simulink model "CaseStudyII_9_Bus"  (R2020a)
settings: Solver=FixedStepAuto  StartTime=0.0  StopTime=Tend  FixedStep=T_s_power  MaxStep=5.0E-5  RelTol=1e-3
values from neighbouring files (symbols this model uses):
  B_s46 = b_s46*Cb    (= 9.5071761847e-07)    [Data_CaseStudyI.m]    (also in Data_CaseStudyII.m; Data_InitialSystem.m)
  B_s54 = b_s54*Cb    (= 1.05902722057e-06)    [Data_CaseStudyI.m]    (also in Data_CaseStudyII.m; Data_InitialSystem.m)
  B_s69 = b_s69*Cb    (= 2.15415764185e-06)    [Data_CaseStudyI.m]    (also in Data_CaseStudyII.m; Data_InitialSystem.m)
  B_s75 = b_s75*Cb    (= 1.84126323577e-06)    [Data_CaseStudyI.m]    (also in Data_CaseStudyII.m; Data_InitialSystem.m)
  B_s87 = b_s87*Cb    (= 8.96562817417e-07)    [Data_CaseStudyI.m]    (also in Data_CaseStudyII.m; Data_InitialSystem.m)
  B_s98 = b_s98*Cb    (= 1.25759482443e-06)    [Data_CaseStudyI.m]    (also in Data_CaseStudyII.m; Data_InitialSystem.m)
  C_dc_DVPP_1_2 = 0.008*(n_DVPP_1_2)    (= 0.8)    [Data_CaseStudyI.m]    (also in Data_CaseStudyII.m)
  C_dc_DVPP_1_3 = 0.008*(n_DVPP_1_3)    (= 0.4)    [Data_CaseStudyI.m]    (also in Data_CaseStudyII.m)
  C_dc_DVPP_3_1 = 0.008*(n_DVPP_3_1)    (= 1.128)    [Data_CaseStudyII.m]
  C_dc_DVPP_3_2 = 0.008*(n_DVPP_3_2)    (= 0.848)    [Data_CaseStudyII.m]
  C_dc_DVPP_3_3 = 0.008*(n_DVPP_3_3)    (= 1.28)    [Data_CaseStudyII.m]
  Dp_DVPP_3_pu = 1/dp_DVPP_3    (= 33.3333333333)    [Data_CaseStudyII.m]
  Dq1_DVPP_3_pu = 100    [Data_CaseStudyII.m]
  fb = 50    [Data_CaseStudyI.m]    (also in Data_CaseStudyII.m; Data_InitialSystem.m)
  HGov_dyn = HGov_delay*H_tr_droop    [Data_CaseStudyI.m]    (also in Data_CaseStudyII.m; Data_InitialSystem.m)
  HTurb_tot = H_water_way    [Data_CaseStudyI.m]    (also in Data_CaseStudyII.m; Data_InitialSystem.m)
  I_m_DVPP_1_2 = 2/3*Sb_DVPP_1_2/V_m_DVPP_1_2    [Data_CaseStudyI.m]    (also in Data_CaseStudyII.m)
  I_m_DVPP_1_3 = 2/3*Sb_DVPP_1_3/V_m_DVPP_1_3    [Data_CaseStudyI.m]    (also in Data_CaseStudyII.m)
  I_m_DVPP_3_1 = 2/3*Sb_DVPP_3_1/V_m_DVPP_3_1    [Data_CaseStudyII.m]
  I_m_DVPP_3_2 = 2/3*Sb_DVPP_3_2/V_m_DVPP_3_2    [Data_CaseStudyII.m]
  I_m_DVPP_3_3 = 2/3*Sb_DVPP_3_3/V_m_DVPP_3_3    [Data_CaseStudyII.m]
  i_star_max = 1.3    [Data_CaseStudyI.m]    (also in Data_CaseStudyII.m)
  iabc_DVPP_1_2_0 = T0*idq0_DVPP_1_2    [Data_CaseStudyI.m]    (also in Data_CaseStudyII.m)
  iabc_DVPP_1_3_0 = T0*idq0_DVPP_1_3    [Data_CaseStudyI.m]    (also in Data_CaseStudyII.m)
  iabc_DVPP_3_1_0 = T0*idq0_DVPP_3_1    [Data_CaseStudyII.m]
  iabc_DVPP_3_2_0 = T0*idq0_DVPP_3_2    [Data_CaseStudyII.m]
  iabc_DVPP_3_3_0 = T0*idq0_DVPP_3_3    [Data_CaseStudyII.m]
  K2_DVPP_1 = [-0.0221795494247 -1.60799665656 0.160449825826 -2.94803557381 -11.8081988371 -9.75170960256 0.00463021906909 -49.1667298155]    [ControlGains_DVPP1.mat]
  K3_DVPP_1 = [-0.0591512752956 -1.61493903379 -27.2946107927 -16.2119211358 -14.3657419818 2.05688388773 -2.27328406162 0.146700393037 -150.920793597]    [ControlGains_DVPP1.mat]
  k_dc_DVPP_1_2 = eta_DVPP_1_2/(Vdc_n_DVPP_1_2*m_p_DVPP_1_2)    [Data_CaseStudyI.m]    (also in Data_CaseStudyII.m)
  k_dc_DVPP_1_3 = eta_DVPP_1_3/(Vdc_n_DVPP_1_3*m_p_DVPP_1_3)    [Data_CaseStudyI.m]    (also in Data_CaseStudyII.m)
  k_dc_DVPP_3_1 = eta_DVPP_3_1/(Vdc_n_DVPP_3_1*m_p_DVPP_3_1)    [Data_CaseStudyII.m]
  k_dc_DVPP_3_2 = eta_DVPP_3_2/(Vdc_n_DVPP_3_2*m_p_DVPP_3_2)    [Data_CaseStudyII.m]
  k_dc_DVPP_3_3 = eta_DVPP_3_3/(Vdc_n_DVPP_3_3*m_p_DVPP_3_3)    [Data_CaseStudyII.m]
  ki_i_pu = 1.19    [Data_CaseStudyI.m]    (also in Data_CaseStudyII.m)
  ki_pll = 1700    [Data_CaseStudyI.m]    (also in Data_CaseStudyII.m)
  ki_q_pu = 0.005    [Data_CaseStudyI.m]    (also in Data_CaseStudyII.m)
  kp_i_pu = 0.73    [Data_CaseStudyI.m]    (also in Data_CaseStudyII.m)
  kp_pll = 150    [Data_CaseStudyI.m]    (also in Data_CaseStudyII.m)
  kp_q_pu = 0.05    [Data_CaseStudyI.m]    (also in Data_CaseStudyII.m)
  L1_DVPP_1_2_pu = 0.0186/m_DVPP_1_2    (= 0.000372)    [Data_CaseStudyI.m]    (also in Data_CaseStudyII.m)
  L1_DVPP_1_3_pu = 0.0186/m_DVPP_1_3    (= 0.000744)    [Data_CaseStudyI.m]    (also in Data_CaseStudyII.m)
  L1_DVPP_3_1_pu = 0.0186/m_DVPP_3_1    (= 0.000263829787234)    [Data_CaseStudyII.m]
  L1_DVPP_3_2_pu = 0.0186/m_DVPP_3_2    (= 0.000350943396226)    [Data_CaseStudyII.m]
  L1_DVPP_3_3_pu = 0.0186/m_DVPP_3_3    (= 0.0002325)    [Data_CaseStudyII.m]
  l1_MVHV1 = 0    [Data_CaseStudyI.m]    (also in Data_CaseStudyII.m; Data_InitialSystem.m)
  l1_MVHV2 = 0    [Data_CaseStudyI.m]    (also in Data_CaseStudyII.m; Data_InitialSystem.m)
  l1_MVHV3 = 0    [Data_CaseStudyI.m]    (also in Data_CaseStudyII.m; Data_InitialSystem.m)
  L2_DVPP_1_2_pu = L1_DVPP_1_2_pu    (= 0.000372)    [Data_CaseStudyI.m]    (also in Data_CaseStudyII.m)
  L2_DVPP_1_3_pu = L1_DVPP_1_3_pu    (= 0.000744)    [Data_CaseStudyI.m]    (also in Data_CaseStudyII.m)
  L2_DVPP_3_1_pu = L1_DVPP_3_1_pu    (= 0.000263829787234)    [Data_CaseStudyII.m]
  L2_DVPP_3_2_pu = L1_DVPP_3_2_pu    (= 0.000350943396226)    [Data_CaseStudyII.m]
  L2_DVPP_3_3_pu = L1_DVPP_3_3_pu    (= 0.0002325)    [Data_CaseStudyII.m]
  l2_MVHV1 = l_s14    (= 0.0576)    [Data_CaseStudyI.m]    (also in Data_CaseStudyII.m; Data_InitialSystem.m)
  l2_MVHV2 = l_s72    (= 0.0625)    [Data_CaseStudyI.m]    (also in Data_CaseStudyII.m; Data_InitialSystem.m)
  l2_MVHV3 = l_s39    (= 0.0586)    [Data_CaseStudyI.m]    (also in Data_CaseStudyII.m; Data_InitialSystem.m)
  l_f_DVPP_1_2 = L_f_DVPP_1_2*w_b/Zb_DVPP_1_2    [Data_CaseStudyI.m]    (also in Data_CaseStudyII.m)
  L_f_DVPP_1_2 = (1/(n_DVPP_1_2))*600*10^-6    (= 6e-06)    [Data_CaseStudyI.m]    (also in Data_CaseStudyII.m)
  l_f_DVPP_1_3 = L_f_DVPP_1_3*w_b/Zb_DVPP_1_3    [Data_CaseStudyI.m]    (also in Data_CaseStudyII.m)
  L_f_DVPP_1_3 = (1/(n_DVPP_1_3))*600*10^-6    (= 1.2e-05)    [Data_CaseStudyI.m]    (also in Data_CaseStudyII.m)
  l_f_DVPP_3_1 = L_f_DVPP_3_1*w_b/Zb_DVPP_3_1    [Data_CaseStudyII.m]
  L_f_DVPP_3_1 = (1/(n_DVPP_3_1))*600*10^-6    (= 4.25531914894e-06)    [Data_CaseStudyII.m]
  l_f_DVPP_3_2 = L_f_DVPP_3_2*w_b/Zb_DVPP_3_2    [Data_CaseStudyII.m]
  L_f_DVPP_3_2 = (1/(n_DVPP_3_2))*600*10^-6    (= 5.66037735849e-06)    [Data_CaseStudyII.m]
  l_f_DVPP_3_3 = L_f_DVPP_3_3*w_b/Zb_DVPP_3_3    [Data_CaseStudyII.m]
  L_f_DVPP_3_3 = (1/(n_DVPP_3_3))*600*10^-6    (= 3.75e-06)    [Data_CaseStudyII.m]
  L_s46 = l_s46*Lb    (= 0.154915055408)    [Data_CaseStudyI.m]    (also in Data_CaseStudyII.m; Data_InitialSystem.m)
  L_s54 = l_s54*Lb    (= 0.143128040323)    [Data_CaseStudyI.m]    (also in Data_CaseStudyII.m; Data_InitialSystem.m)
  L_s69 = l_s69*Lb    (= 0.286256080645)    [Data_CaseStudyI.m]    (also in Data_CaseStudyII.m; Data_InitialSystem.m)
  L_s75 = l_s75*Lb    (= 0.271101346964)    [Data_CaseStudyI.m]    (also in Data_CaseStudyII.m; Data_InitialSystem.m)
  L_s87 = l_s87*Lb    (= 0.12123786945)    [Data_CaseStudyI.m]    (also in Data_CaseStudyII.m; Data_InitialSystem.m)
  L_s98 = l_s98*Lb    (= 0.16973301723)    [Data_CaseStudyI.m]    (also in Data_CaseStudyII.m; Data_InitialSystem.m)
  LPV_K1_DVPP_3 = [0.014519129833 -1.24253756746e-17 -0.00331576987938 -1.41950397655e-17 -0.00331577010739 -1.6423216922e-19 0.0145191298795 1.47256053017e-18 1.92456501739e-17 0.00968260817745 7.5102914291e-19 0.0096826081765 ... (80 elements, 8x10)]    [ControlGains_DVPP3_LPV.mat]
  LPV_K2_DVPP_3 = [0.0299413265511 -2.72480441208e-16 -0.00563144274341 -6.63344905835e-17 -0.00563144273182 -1.08918556426e-16 0.0299413268326 -1.32404731664e-16 -4.78559537004e-17 -0.00914230292149 -8.50409089014e-21 -0.00914230292147 ... (80 elements, 8x10)]    [ControlGains_DVPP3_LPV.mat]
  LPV_K3_DVPP_3 = [-0.0173301370849 5.00398589077e-17 -0.0636125194304 3.31757376688e-17 -0.0636125164794 5.41726806116e-17 -0.017330137145 2.43427565927e-17 -0.0400570975704 -5.68753124238e-17 -0.0574012283733 2.45717741258e-17 ... (192 elements, 16x12)]    [ControlGains_DVPP3_LPV.mat]
  Mp_DVPP_3_pu = 13    [Data_CaseStudyII.m]
  P_L = pL*Sb    (= 300000000)    [Data_CaseStudyI.m]    (also in Data_CaseStudyII.m; Data_InitialSystem.m)
  p_set_bus1 = P_set_bus1/SbSG1    (= 0.731707317073)    [Data_CaseStudyI.m]    (also in Data_CaseStudyII.m; Data_InitialSystem.m)
  p_set_bus2 = P_set_bus2/SbSG2    (= 0.756707317073)    [Data_CaseStudyI.m]    (also in Data_CaseStudyII.m; Data_InitialSystem.m)
  Pb_DVPP_3_1 = 37e6    (= 37000000)    [Data_CaseStudyII.m]
  Pb_DVPP_3_2 = 28e6    (= 28000000)    [Data_CaseStudyII.m]
  Pb_DVPP_3_3 = 0e6    (= 0)    [Data_CaseStudyII.m]
  pset_DVPP_1_1 = P_set_bus1/SbSG1    (= 0.731707317073)    [Data_CaseStudyI.m]    (also in Data_CaseStudyII.m)
  pset_DVPP_1_2 = 0    [Data_CaseStudyI.m]    (also in Data_CaseStudyII.m)
  pset_DVPP_1_3 = 0    [Data_CaseStudyI.m]    (also in Data_CaseStudyII.m)
  pset_DVPP_3_1 = (0.6*P_set_bus3)/Sb_DVPP_3_1    (= 0.398546964193)    [Data_CaseStudyII.m]
  pset_DVPP_3_2 = (0.4*P_set_bus3)/Sb_DVPP_3_2    (= 0.353428439945)    [Data_CaseStudyII.m]
  pset_DVPP_3_3 = 0    [Data_CaseStudyII.m]
  Q_L = qL*Sb    (= 82500000)    [Data_CaseStudyI.m]    (also in Data_CaseStudyII.m; Data_InitialSystem.m)
  qset_DVPP_1_2 = 0    [Data_CaseStudyI.m]    (also in Data_CaseStudyII.m)
  qset_DVPP_1_3 = 0    [Data_CaseStudyI.m]    (also in Data_CaseStudyII.m)
  qset_DVPP_3_1 = 0    [Data_CaseStudyII.m]
  qset_DVPP_3_2 = 0    [Data_CaseStudyII.m]
  qset_DVPP_3_3 = 0    [Data_CaseStudyII.m]
  R1_DVPP_1_2_pu = 0.00734/m_DVPP_1_2    (= 0.0001468)    [Data_CaseStudyI.m]    (also in Data_CaseStudyII.m)
  R1_DVPP_1_3_pu = 0.00734/m_DVPP_1_3    (= 0.0002936)    [Data_CaseStudyI.m]    (also in Data_CaseStudyII.m)
  R1_DVPP_3_1_pu = 0.00734/m_DVPP_3_1    (= 0.000104113475177)    [Data_CaseStudyII.m]
  R1_DVPP_3_2_pu = 0.00734/m_DVPP_3_2    (= 0.000138490566038)    [Data_CaseStudyII.m]
  R1_DVPP_3_3_pu = 0.00734/m_DVPP_3_3    (= 9.175e-05)    [Data_CaseStudyII.m]
  r1_MVHV1 = 1e-6    (= 1e-06)    [Data_CaseStudyI.m]    (also in Data_CaseStudyII.m; Data_InitialSystem.m)
  r1_MVHV2 = 1e-6    (= 1e-06)    [Data_CaseStudyI.m]    (also in Data_CaseStudyII.m; Data_InitialSystem.m)
  r1_MVHV3 = 1e-6    (= 1e-06)    [Data_CaseStudyI.m]    (also in Data_CaseStudyII.m; Data_InitialSystem.m)
  R2_DVPP_1_2_pu = R1_DVPP_1_2_pu    (= 0.0001468)    [Data_CaseStudyI.m]    (also in Data_CaseStudyII.m)
  R2_DVPP_1_3_pu = R1_DVPP_1_3_pu    (= 0.0002936)    [Data_CaseStudyI.m]    (also in Data_CaseStudyII.m)
  R2_DVPP_3_1_pu = R1_DVPP_3_1_pu    (= 0.000104113475177)    [Data_CaseStudyII.m]
  R2_DVPP_3_2_pu = R1_DVPP_3_2_pu    (= 0.000138490566038)    [Data_CaseStudyII.m]
  R2_DVPP_3_3_pu = R1_DVPP_3_3_pu    (= 9.175e-05)    [Data_CaseStudyII.m]
  r2_MVHV1 = 1e-6    (= 1e-06)    [Data_CaseStudyI.m]    (also in Data_CaseStudyII.m; Data_InitialSystem.m)
  r2_MVHV2 = 1e-6    (= 1e-06)    [Data_CaseStudyI.m]    (also in Data_CaseStudyII.m; Data_InitialSystem.m)
  r2_MVHV3 = 1e-6    (= 1e-06)    [Data_CaseStudyI.m]    (also in Data_CaseStudyII.m; Data_InitialSystem.m)
  R_dc_DVPP_1_2 = (Vdc_n_DVPP_1_2/(0.05*(Sb_DVPP_1_2)/Vdc_n_DVPP_1_2))    [Data_CaseStudyI.m]    (also in Data_CaseStudyII.m)
  R_dc_DVPP_1_3 = (Vdc_n_DVPP_1_3/(0.05*(Sb_DVPP_1_3)/Vdc_n_DVPP_1_3))    [Data_CaseStudyI.m]    (also in Data_CaseStudyII.m)
  R_dc_DVPP_3_1 = (Vdc_n_DVPP_3_1/(0.05*(Sb_DVPP_3_1)/Vdc_n_DVPP_3_1))    [Data_CaseStudyII.m]
  R_dc_DVPP_3_2 = (Vdc_n_DVPP_3_2/(0.05*(Sb_DVPP_3_2)/Vdc_n_DVPP_3_2))    [Data_CaseStudyII.m]
  R_dc_DVPP_3_3 = (Vdc_n_DVPP_3_3/(0.05*(Sb_DVPP_3_3)/Vdc_n_DVPP_3_3))    [Data_CaseStudyII.m]
  r_f_DVPP_1_2 = R_f_DVPP_1_2/Zb_DVPP_1_2    [Data_CaseStudyI.m]    (also in Data_CaseStudyII.m)
  R_f_DVPP_1_2 = 0.02/n_DVPP_1_2    (= 0.0002)    [Data_CaseStudyI.m]    (also in Data_CaseStudyII.m)
  r_f_DVPP_1_3 = R_f_DVPP_1_3/Zb_DVPP_1_3    [Data_CaseStudyI.m]    (also in Data_CaseStudyII.m)
  R_f_DVPP_1_3 = 0.02/n_DVPP_1_3    (= 0.0004)    [Data_CaseStudyI.m]    (also in Data_CaseStudyII.m)
  r_f_DVPP_3_1 = R_f_DVPP_3_1/Zb_DVPP_3_1    [Data_CaseStudyII.m]
  ... (+104 more)
undefined symbols (not defined in the file or in its folder): A, B, C, Continuous, Dd, Efd0, gcbh, i_dc, Ka, Kf, p2set, SbSM2, sps_rtmsupport, spsST1AModel, Ta, Tb, Tb1, Tc, Tc1, Tf, VA0, VAmax, VAmin, VImax, VImin, VRmax, VRmin
libraries: powerlib x95, powerlib_meascontrol x41, cstblocks x15, sps_avr x1, simulink_extras x1, simulink x1
(part 5 of 5)

== system CaseStudyII_9_Bus/Supercapacitor/Power Controllers/Reactive Power Controller PI-droop control ==
  Q_abc : Inport
  Qset : Inport  Port=2
  Gain : Gain  Gain=kp_q_pu
  Gain1 : Gain  Gain=ki_q_pu
  Integrator1 : Integrator  InitialCondition=xq0_DVPP_1_3_pu
  Sum : Sum  Inputs=-+
  Sum1 : Sum
  i_star_q : Outport
  wires:
  Q_abc/1 -> Sum/2
  Qset/1 -> Sum/1
  Sum/1 -> Integrator1/1, Gain/1
  Gain/1 -> Sum1/1
  Gain1/1 -> Sum1/2
  Integrator1/1 -> Gain1/1
  Sum1/1 -> i_star_q/1

== system CaseStudyII_9_Bus/Synchronous Machine 2 reheat steam turbine/ST1A Excitation System/Model ==
  note: Efd0
  note: Efd0
  note: VA0/Ka
  note: VA0/Ka
  note: Vt.VRmin
  note: VA0/Ka
  note: Efd0
  note: 0
  note: Vt0
  note: Vt.VRmax-Kc.Ifd
  note: Main Regulator
      | Ka/(Ta.s+1)
  note: VImax
  note: Initial values are shown in blue
  note: Vt0
  note: __
      |              /
      |           /
      |         /
      |       /
      | __/
  note: Limits VImin, VImax
  note: VAmax
  note: VAmin
  note: VA0/Ka
  note: KLR*(Ifd-ILR)
  note: VA0=Efd0+KLR*(Ifd-ILR)
  note: VA0
  note: Vt0
  Vref : Inport
  Vt : Inport  Port=2
  Ifd : Inport  Port=3
  Vstab : Inport  Port=4
  Damping Filter Kf.s/(Tf.s+1) : Subsystem  mask(Transfer Function with Initial Outputs){N=[Kf 0], D=[Tf 1], Y0=0, U0=Efd0}
      mask prompts: N "Numerator:"; D "Denominator:"; Y0 "Initial output:"; U0 "Initial input:"
      mask help: Vector expressions for numerator, and denominator. Coefficients are in descending powers of s.
      mask init:
      | [A,B,C,Dd]=tf2ss(N,D);
      | if (isempty(Y0));
      |     [m,n]=size(C);
      |     Y0=zeros(1,m); 
      | end; 
      | if (isempty(U0));
      |     [m,p]=size(B);
      |     U0=zeros(1,p);
      | end;
      | X0=getxo(A,B,C,Dd,U0,Y0,0);
      mask Help: Specify the initial output for the transfer function.  An optimization routine attempts to determine the appropriate initial states so that the specified initial output is achieved.  For more details, see the m-file getxo.m
      mask Display: dpoly(N,D,'s')
  ILR : Constant  Value=ILR
  KLR : Gain  Gain=KLR  SaturateOnIntegerOverflow=on  OutDataTypeStr=Inherit: Same as input  ParamDataTypeStr=Inherit: Same as input
  Low Pass Filter 1/(Tr.s+1) : simulink_extras/Additional Linear/Transfer Fcn (with initial outputs)  N=1  D=[Tr 1]  Y0=Vt0  U0=Vt0
  Subsystem : Subsystem
      mask Display: plot([0.15 0.85],[.5 .5],[.5 .5],[0.05 0.95],0.15+0.7*[0 .25 .75 1],0.05+0.9*[.25 .25 .75 .75]);
  Subtract : Sum  Inputs=+-
  Sum : Sum  Inputs=++-+-  InputSameDT=on  SaturateOnIntegerOverflow=on  OutDataTypeStr=Inherit: Same as first input
  Sum1 : Sum  Inputs=|+-  InputSameDT=on  SaturateOnIntegerOverflow=on  OutDataTypeStr=Inherit: Same as first input
  Sum2 : Sum  Inputs=|+-  InputSameDT=on  SaturateOnIntegerOverflow=on  OutDataTypeStr=Inherit: Same as first input
  Transient Gain Reduction (Tc.s+1).(Tc1.s+1) ----------------------- (Tb.s+1).(Tb1.s+1) : Subsystem  mask(Transfer Function with Initial Outputs){N=[Tc*Tc1 Tc+Tc1 1], D=[Tb*Tb1 Tb+Tb1 1], Y0=VA0/Ka, U0=VA0/Ka}
      mask prompts: N "Numerator:"; D "Denominator:"; Y0 "Initial output:"; U0 "Initial input:"
      mask help: Vector expressions for numerator, and denominator. Coefficients are in descending powers of s.
      mask init:
      | [A,B,C,Dd]=tf2ss(N,D);if (isempty(Y0));[m,n]=size(A);X0=zeros(1,m); end; if (isempty(U0));[m,p]=size(B);U0=zeros(1,p);end;
      |  if isempty(A),  X0=[]; else ,X0=getxo(A,B,C,Dd,U0,Y0,0); end
      mask Help: Specify the initial output for the transfer function.  An optimization routine attempts to determine the appropriate initial states so that the specified initial output is achieved.  For more details, see the m-file getxo.m
      mask Display: dpoly(N,D,'s')
  VA0/Ka : Constant  Value=VA0/Ka
  VImin : Saturate  UpperLimit=VImax  LowerLimit=VImin
  VImin2 : Saturate  UpperLimit=inf  LowerLimit=0
  Vaminmax : Subsystem  mask{Ka=Ka, Ta=Ta, VAminmax=[VAmin VAmax], X0=VA0}
      mask prompts: Ka "Voltage regulator gain Ka:"; Ta "Voltage regulator time constant Ta(s):"; VAminmax "Voltage regulator internal limits [VAmin(pu) VAmax(pu)]:"; X0 "Initial conditions:"
      mask init:
      | VAmin=VAminmax(1);VAmax=VAminmax(2);
      mask Display: dpoly([Ka],[Ta 1],'s')
  Efd : Outport
  wires:
  Ifd/1 -> Sum1/1, Subsystem/3(Ifd)
  Subsystem/1(Efd1) -> Efd/1  "Efd"
  Vt/1 -> Low Pass Filter 1/(Tr.s+1)/1  "Vt"
  Vaminmax/1(y) -> Sum2/1  "VA"
  Sum/1 -> VImin/1
  Sum1/1 -> KLR/1
  ILR/1 -> Sum1/2
  Sum2/1 -> Damping Filter Kf.s/(Tf.s+1)/1(In1), Subsystem/1(Efd)  "Efd"
  Transient Gain Reduction (Tc.s+1).(Tc1.s+1) ----------------------- (Tb.s+1).(Tb1.s+1)/1(Out1) -> Vaminmax/1(u)
  KLR/1 -> VImin2/1
  VA0/Ka/1 -> Sum/2
  Low Pass Filter 1/(Tr.s+1)/1 -> Subtract/2, Subsystem/2(Vt)  "Vt"
  VImin2/1 -> Sum2/2
  Damping Filter Kf.s/(Tf.s+1)/1(Out1) -> Sum/5  "Vf"
  VImin/1 -> Transient Gain Reduction (Tc.s+1).(Tc1.s+1) ----------------------- (Tb.s+1).(Tb1.s+1)/1(In1)  "VI"
  Vstab/1 -> Sum/4
  Vref/1 -> Subtract/1
  Subtract/1 -> Sum/1

== system CaseStudyII_9_Bus/Wind /PLL/Subsystem ==
  Vabc : Inport  PortDimensions=3
  Constant : Constant  Value=2*pi*50
  Demux2 : Demux  Outputs=3
  Divide : Product  Inputs=/*
  First-Order Filter : powerlib_meascontrol/Filters/First-Order Filter  FilterType=Lowpass  Tc=0.081  Ts=0  Initialize=on  Vac_Init=[0, 0, fb]  Vdc_Init=0  PlotResponse=off  FreqRange="[0,  200,  1]"
  Gain : Gain  Gain=kp_pll
  Gain1 : Gain  Gain=ki_pll
  Gain10 : Gain  Gain=1/2/pi  SaturateOnIntegerOverflow=on  OutDataTypeStr=Inherit: Same as input  ParamDataTypeStr=Inherit: Same as input
  Integrator : Integrator
  Integrator1 : Integrator  InitialCondition=xpll0_pu
  Memory : Memory  InitialCondition=fb
  Selector : Selector  InputPortWidth=3  IndexOptions=Index vector (dialog)  Indices=2  OutputSizes=1
  Sqrt2 : Sqrt  SaturateOnIntegerOverflow=on
  Sum : Sum
  Sum1 : Sum  Inputs=++|
  Sum2 : Sum  Inputs=+++  InputSameDT=on  SaturateOnIntegerOverflow=on  OutDataTypeStr=Inherit: Same as first input
  abc to dq0 : powerlib_meascontrol/Transformations/abc to dq0  Alignment=90 degrees behind phase A axis
      settings: SourceProductBaseCode=MT,PS
  d²2 : Product  InputSameDT=on  RndMeth=Zero  SaturateOnIntegerOverflow=on  OutDataTypeStr=Inherit: Same as first input
  q²4 : Product  InputSameDT=on  RndMeth=Zero  SaturateOnIntegerOverflow=on  OutDataTypeStr=Inherit: Same as first input
  q²5 : Product  InputSameDT=on  RndMeth=Zero  SaturateOnIntegerOverflow=on  OutDataTypeStr=Inherit: Same as first input
  Freq : Outport  VectorParamsAs1DForOutWhenUnconnected=off
  wt : Outport  Port=2  VectorParamsAs1DForOutWhenUnconnected=off
  wires:
  Vabc/1 -> abc to dq0/1
  Integrator/1 -> wt/1, abc to dq0/2
  Memory/1 -> Freq/1
  Gain/1 -> Sum/1
  Gain1/1 -> Sum/2
  Integrator1/1 -> Gain1/1
  Demux2/1 -> d²2/1, d²2/2  "d"
  d²2/1 -> Sum2/1
  Demux2/3 -> q²5/1, q²5/2  "0"
  Demux2/2 -> q²4/1, q²4/2  "q"
  Sqrt2/1 -> Divide/1
  Sum2/1 -> Sqrt2/1
  q²5/1 -> Sum2/3
  abc to dq0/1 -> Demux2/1, Selector/1
  q²4/1 -> Sum2/2
  Selector/1 -> Divide/2  "Vq"
  Divide/1 -> Integrator1/1, Gain/1
  Gain10/1 -> First-Order Filter/1
  First-Order Filter/1 -> Memory/1
  Constant/1 -> Sum1/1
  Sum/1 -> Sum1/2  "W"
  Sum1/1 -> Integrator/1, Gain10/1  "W"

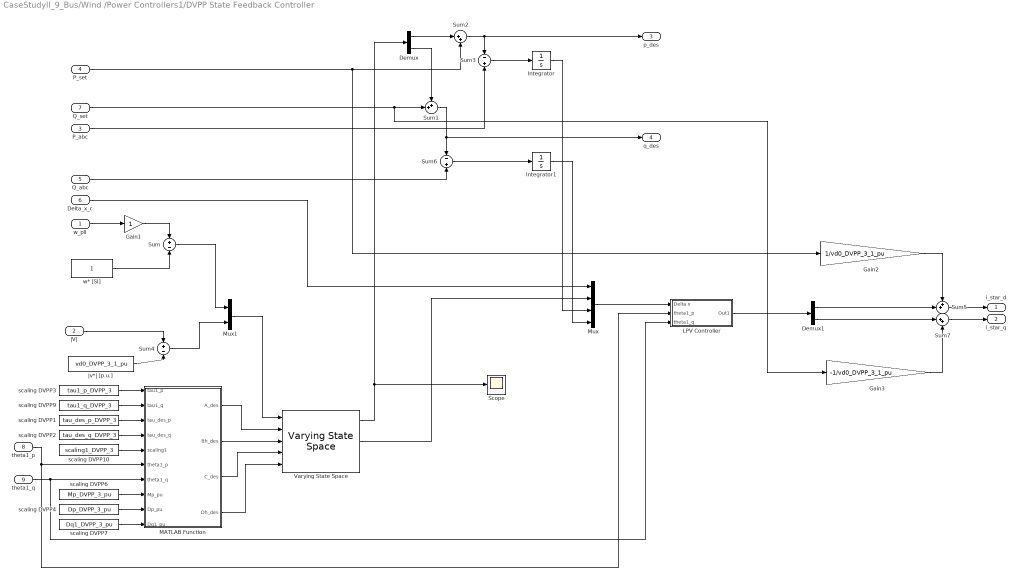
== system CaseStudyII_9_Bus/Wind /Power Controllers1/DVPP State Feedback Controller ==
  w_pll : Inport
  "|V| " : Inport  Port=2
  P_abc : Inport  Port=3
  P_set : Inport  Port=4
  Q_abc : Inport  Port=5
  Delta_x_c : Inport  Port=6
  Q_set : Inport  Port=7
  theta1_p : Inport  Port=8
  theta1_q : Inport  Port=9
  Demux : Demux  Outputs=2
  Demux1 : Demux  Outputs=2
  Gain1 : Gain
  Gain2 : Gain  Gain=1/vd0_DVPP_3_1_pu
  Gain3 : Gain  Gain=-1/vd0_DVPP_3_1_pu
  Integrator : Integrator
  Integrator1 : Integrator
  LPV Controller : Subsystem
  MATLAB Function : MATLAB Function  TreatAsAtomicUnit=on
  Mux : Mux
  Mux1 : Mux  Inputs=2
  Scope : Scope
  Sum : Sum  Inputs=+-
  Sum1 : Sum  Inputs=++|
  Sum2 : Sum  Inputs=|++
  Sum3 : Sum  Inputs=-+
  Sum4 : Sum  Inputs=+-
  Sum5 : Sum  Inputs=++|
  Sum6 : Sum  Inputs=-+
  Sum7 : Sum  Inputs=|++
  Varying State Space : cstblocks/Linear Parameter Varying/Varying State Space  x0=0  xNames=''  OutputX=on  OutputDX=on
  scaling DVPP1 : Constant  Value=tau_des_p_DVPP_3
  scaling DVPP10 : Constant  Value=scaling1_DVPP_3
  scaling DVPP2 : Constant  Value=tau_des_q_DVPP_3
  scaling DVPP3 : Constant  Value=tau1_p_DVPP_3
  scaling DVPP4 : Constant  Value=Dp_DVPP_3_pu
  scaling DVPP6 : Constant  Value=Mp_DVPP_3_pu
  scaling DVPP7 : Constant  Value=Dq1_DVPP_3_pu
  scaling DVPP9 : Constant  Value=tau1_q_DVPP_3
  w* [SI] : Constant
  |v*| [p.u.] : Constant  Value=vd0_DVPP_3_1_pu
  i_star_d : Outport
  i_star_q : Outport  Port=2
  p_des : Outport  Port=3
  q_des : Outport  Port=4
  wires:
  Mux/1 -> LPV Controller/1(Delta x)
  Sum3/1 -> Integrator/1
  "|V| "/1 -> Sum4/1
  |v*| [p.u.]/1 -> Sum4/2
  w_pll/1 -> Gain1/1
  w* [SI]/1 -> Sum/2
  Sum/1 -> Mux1/1
  Mux1/1 -> Varying State Space/1
  Varying State Space/1 -> Demux/1, Scope/1
  P_abc/1 -> Sum3/2
  Q_abc/1 -> Sum6/2
  Sum6/1 -> Integrator1/1
  Integrator/1 -> Mux/3
  Integrator1/1 -> Mux/4
  Varying State Space/2 -> Mux/2
  Delta_x_c/1 -> Mux/1
  LPV Controller/1(Out1) -> Demux1/1
  Gain1/1 -> Sum/1
  Sum4/1 -> Mux1/2
  Q_set/1 -> Gain3/1, Sum1/2
  Demux/2 -> Sum1/1
  Sum1/1 -> q_des/1, Sum6/1
  Demux/1 -> Sum2/1
  Sum2/1 -> p_des/1, Sum3/1
  P_set/1 -> Gain2/1, Sum2/2
  Demux1/1 -> Sum5/2
  Sum5/1 -> i_star_d/1
  Gain2/1 -> Sum5/1
  Sum7/1 -> i_star_q/1
  Gain3/1 -> Sum7/2
  Demux1/2 -> Sum7/1
  MATLAB Function/1(A_des) -> Varying State Space/2
  MATLAB Function/2(Bh_des) -> Varying State Space/3
  MATLAB Function/3(C_des) -> Varying State Space/4
  MATLAB Function/4(Dh_des) -> Varying State Space/5
  scaling DVPP3/1 -> MATLAB Function/1(tau1_p)
  scaling DVPP9/1 -> MATLAB Function/2(tau1_q)
  scaling DVPP1/1 -> MATLAB Function/3(tau_des_p)
  scaling DVPP2/1 -> MATLAB Function/4(tau_des_q)
  scaling DVPP10/1 -> MATLAB Function/5(scaling1)
  scaling DVPP6/1 -> MATLAB Function/8(Mp_pu)
  scaling DVPP4/1 -> MATLAB Function/9(Dp_pu)
  scaling DVPP7/1 -> MATLAB Function/10(Dq1_pu)
  theta1_p/1 -> LPV Controller/2(theta1_p), MATLAB Function/6(theta1_p)
  theta1_q/1 -> LPV Controller/3(theta1_q), MATLAB Function/7(theta1_q)

== system CaseStudyII_9_Bus/PV/Power Controllers/DVPP State Feedback Controller/LPV Controller ==
  Delta x : Inport
  theta2_p : Inport  Port=2
  theta2_q : Inport  Port=3
  Add : Sum  Inputs=++++
  Constant : Constant  Value=theta2_p_1
  Constant1 : Constant  Value=theta2_p_2
  Constant2 : Constant  Value=theta2_q_2
  Constant3 : Constant  Value=theta2_q_1
  Gain : Gain  Gain=LPV_K2_DVPP_3(1:2,:)
  Gain1 : Gain  Gain=LPV_K2_DVPP_3(3:4,:)
  Gain2 : Gain  Gain=LPV_K2_DVPP_3(5:6,:)
  Gain3 : Gain  Gain=LPV_K2_DVPP_3(7:8,:)
  MATLAB Function : MATLAB Function  TreatAsAtomicUnit=on
  Reshape : Reshape  OutputDimensionality=Customize  OutputDimensions=[2,10]
  Reshape1 : Reshape  OutputDimensionality=Customize  OutputDimensions=[10,1]
  multiply : Product  Multiplication=Matrix(*)
  Out1 : Outport
  wires:
  MATLAB Function/1(lambda1) -> Gain/1
  MATLAB Function/2(lambda2) -> Gain1/1
  Gain/1 -> Add/1
  Gain1/1 -> Add/2
  multiply/1 -> Out1/1
  Add/1 -> Reshape/1
  Delta x/1 -> Reshape1/1
  theta2_p/1 -> MATLAB Function/1(theta2_p)
  theta2_q/1 -> MATLAB Function/2(theta2_q)
  Constant/1 -> MATLAB Function/3(theta2_p_1)
  Constant1/1 -> MATLAB Function/4(theta2_p_2)
  Constant3/1 -> MATLAB Function/5(theta2_q_1)
  Constant2/1 -> MATLAB Function/6(theta2_q_2)
  Gain2/1 -> Add/3
  MATLAB Function/3(lambda3) -> Gain2/1
  MATLAB Function/4(lambda4) -> Gain3/1
  Gain3/1 -> Add/4
  Reshape/1 -> multiply/1
  Reshape1/1 -> multiply/2

== system CaseStudyII_9_Bus/STATCOM with Battery/Power Controllers1/DVPP State Feedback Controller/LPV Controller ==
  Delta x : Inport
  theta1_p : Inport  Port=2
  theta2_p : Inport  Port=3
  theta3_q : Inport  Port=4
  Add : Sum  Inputs=++++++++
  Constant : Constant  Value=theta2_p_1
  Constant1 : Constant  Value=theta2_p_2
  Constant2 : Constant  Value=theta3_q_2
  Constant3 : Constant  Value=theta3_q_1
  Constant4 : Constant  Value=theta1_p_1
  Constant5 : Constant  Value=theta1_p_2
  Gain : Gain  Gain=LPV_K3_DVPP_3(1:2,:)
  Gain1 : Gain  Gain=LPV_K3_DVPP_3(3:4,:)
  Gain2 : Gain  Gain=LPV_K3_DVPP_3(5:6,:)
  Gain3 : Gain  Gain=LPV_K3_DVPP_3(7:8,:)
  Gain4 : Gain  Gain=LPV_K3_DVPP_3(9:10,:)
  Gain5 : Gain  Gain=LPV_K3_DVPP_3(11:12,:)
  Gain6 : Gain  Gain=LPV_K3_DVPP_3(13:14,:)
  Gain7 : Gain  Gain=LPV_K3_DVPP_3(15:16,:)
  MATLAB Function : MATLAB Function  TreatAsAtomicUnit=on
  Reshape : Reshape  OutputDimensionality=Customize  OutputDimensions=[2,12]
  Reshape1 : Reshape  OutputDimensionality=Customize  OutputDimensions=[12,1]
  multiply : Product  Multiplication=Matrix(*)
  Out1 : Outport
  wires:
  multiply/1 -> Out1/1
  Add/1 -> Reshape/1
  Delta x/1 -> Reshape1/1
  Constant2/1 -> MATLAB Function/9(theta3_q_2)
  Constant3/1 -> MATLAB Function/8(theta3_q_1)
  Constant1/1 -> MATLAB Function/7(theta2_p_2)
  Constant/1 -> MATLAB Function/6(theta2_p_1)
  Constant4/1 -> MATLAB Function/4(theta1_p_1)
  Constant5/1 -> MATLAB Function/5(theta1_p_2)
  theta1_p/1 -> MATLAB Function/1(theta1_p)
  theta2_p/1 -> MATLAB Function/2(theta2_p)
  theta3_q/1 -> MATLAB Function/3(theta3_q)
  MATLAB Function/1(lambda1) -> Gain/1
  MATLAB Function/2(lambda2) -> Gain1/1
  Gain/1 -> Add/1
  Gain1/1 -> Add/2
  MATLAB Function/3(lambda3) -> Gain2/1
  Gain2/1 -> Add/3
  MATLAB Function/4(lambda4) -> Gain3/1
  Gain3/1 -> Add/4
  MATLAB Function/5(lambda5) -> Gain4/1
  MATLAB Function/6(lambda6) -> Gain5/1
  MATLAB Function/7(lambda7) -> Gain6/1
  MATLAB Function/8(lambda8) -> Gain7/1
  Gain4/1 -> Add/5
  Gain5/1 -> Add/6
  Gain6/1 -> Add/7
  Gain7/1 -> Add/8
  Reshape/1 -> multiply/1
  Reshape1/1 -> multiply/2

== system CaseStudyII_9_Bus/Synchronous Machine 2 reheat steam turbine/ST1A Excitation System/Model/Damping Filter Kf.s//(Tf.s+1) ==
  In1 : Inport
  State Space : StateSpace  A=A  B=B  C=C  D=Dd  InitialCondition=X0
  Out1 : Outport  InitialOutput=0
  wires:
  In1/1 -> State Space/1
  State Space/1 -> Out1/1

== system CaseStudyII_9_Bus/Synchronous Machine 2 reheat steam turbine/ST1A Excitation System/Model/Subsystem ==
  note: Vt.VRmax-Kc.Ifd
  note: Vt.VRmin
  Efd : Inport
  Vt : Inport  Port=2
  Ifd : Inport  Port=3
  Gain2 : Gain  Gain=Kc  SaturateOnIntegerOverflow=on  OutDataTypeStr=Inherit: Same as input  ParamDataTypeStr=Inherit: Same as input
  Gain5 : Gain  Gain=VRmax  SaturateOnIntegerOverflow=on  OutDataTypeStr=Inherit: Same as input  ParamDataTypeStr=Inherit: Same as input
  Gain6 : Gain  Gain=VRmin  SaturateOnIntegerOverflow=on  OutDataTypeStr=Inherit: Same as input  ParamDataTypeStr=Inherit: Same as input
  Saturation Dynamic : simulink/Discontinuities/Saturation Dynamic  OutMin=[]  OutMax=[]  OutDataTypeStr=Inherit: Same as second input  OutDataType=fixdt(1, 16)  OutScaling=2^-10  DoSatur=off
  Sum5 : Sum  Inputs=+-  InputSameDT=on  SaturateOnIntegerOverflow=on  OutDataTypeStr=Inherit: Same as first input
  Efd1 : Outport
  wires:
  Gain2/1 -> Sum5/2
  Ifd/1 -> Gain2/1  "Field current Ifd (pu)"
  Efd/1 -> Saturation Dynamic/2  "Field voltage Efd (pu)"
  Gain6/1 -> Saturation Dynamic/3
  Saturation Dynamic/1 -> Efd1/1
  Gain5/1 -> Sum5/1
  Vt/1 -> Gain6/1, Gain5/1  "Terminal voltage Vt (pu)"
  Sum5/1 -> Saturation Dynamic/1

== system CaseStudyII_9_Bus/Synchronous Machine 2 reheat steam turbine/ST1A Excitation System/Model/Transient Gain Reduction (Tc.s+1).(Tc1.s+1) ----------------------- (Tb.s+1).(Tb1.s+1) ==
  In1 : Inport
  State Space : StateSpace  A=A  B=B  C=C  D=Dd  InitialCondition=X0
  Out1 : Outport  InitialOutput=0
  wires:
  In1/1 -> State Space/1
  State Space/1 -> Out1/1

== system CaseStudyII_9_Bus/Synchronous Machine 2 reheat steam turbine/ST1A Excitation System/Model/Vaminmax ==
  note: VA0/Ka
  note: VA0
  note: VA0
  note: 0
  note: VA0
  u : Inport
  Gain1 : Gain  Gain=1/Ta  SaturateOnIntegerOverflow=on  OutDataTypeStr=Inherit: Same as input  ParamDataTypeStr=Inherit: Same as input
  Gain2 : Gain  Gain=Ka  SaturateOnIntegerOverflow=on  OutDataTypeStr=Inherit: Same as input  ParamDataTypeStr=Inherit: Same as input
  Integrator : Integrator  InitialCondition=VA0  LimitOutput=on  UpperSaturationLimit=VAmax  LowerSaturationLimit=VAmin
  Sum : Sum  Inputs=|+-  InputSameDT=on  SaturateOnIntegerOverflow=on  OutDataTypeStr=Inherit: Same as first input
  y : Outport
  wires:
  u/1 -> Gain2/1
  Sum/1 -> Gain1/1
  Integrator/1 -> y/1, Sum/2
  Gain2/1 -> Sum/1
  Gain1/1 -> Integrator/1

== system CaseStudyII_9_Bus/Wind /Power Controllers1/DVPP State Feedback Controller/LPV Controller ==
  Delta x : Inport
  theta1_p : Inport  Port=2
  theta1_q : Inport  Port=3
  Add : Sum  Inputs=++++
  Constant : Constant  Value=theta1_p_1
  Constant1 : Constant  Value=theta1_p_2
  Constant2 : Constant  Value=theta1_q_2
  Constant3 : Constant  Value=theta1_q_1
  Gain : Gain  Gain=LPV_K1_DVPP_3(1:2,:)
  Gain1 : Gain  Gain=LPV_K1_DVPP_3(3:4,:)
  Gain2 : Gain  Gain=LPV_K1_DVPP_3(5:6,:)
  Gain3 : Gain  Gain=LPV_K1_DVPP_3(7:8,:)
  MATLAB Function : MATLAB Function  TreatAsAtomicUnit=on
  Reshape : Reshape  OutputDimensionality=Customize  OutputDimensions=[2,10]
  Reshape1 : Reshape  OutputDimensionality=Customize  OutputDimensions=[10,1]
  multiply : Product  Multiplication=Matrix(*)
  Out1 : Outport
  wires:
  MATLAB Function/1(lambda1) -> Gain/1
  MATLAB Function/2(lambda2) -> Gain1/1
  Gain/1 -> Add/1
  Gain1/1 -> Add/2
  multiply/1 -> Out1/1
  Add/1 -> Reshape/1
  Delta x/1 -> Reshape1/1
  theta1_p/1 -> MATLAB Function/1(theta1_p)
  theta1_q/1 -> MATLAB Function/2(theta1_q)
  Constant/1 -> MATLAB Function/3(theta1_p_1)
  Constant1/1 -> MATLAB Function/4(theta1_p_2)
  Constant3/1 -> MATLAB Function/5(theta1_q_1)
  Constant2/1 -> MATLAB Function/6(theta1_q_2)
  Gain2/1 -> Add/3
  MATLAB Function/3(lambda3) -> Gain2/1
  MATLAB Function/4(lambda4) -> Gain3/1
  Gain3/1 -> Add/4
  Reshape/1 -> multiply/1
  Reshape1/1 -> multiply/2

== matlab function CaseStudyII_9_Bus/STATCOM with Battery/Power Controllers1/DVPP State Feedback Controller/MATLAB Function ==
  data: tau1_p input; tau2_p input; tau3_p input; tau3_q input; tau_des_p input; tau_des_q input; scaling3 input; theta1_p input; A_des output; Bh_des output; C_des output; Dh_des output; theta2_p input; theta3_q input; Mp_pu input; Dp_pu input; Dq1_pu input
function [A_des, Bh_des, C_des, Dh_des] = fcn(tau1_p,tau2_p,tau3_p,tau3_q,tau_des_p,tau_des_q, scaling3,theta1_p, theta2_p, theta3_q, Mp_pu, Dp_pu, Dq1_pu)

A_des = zeros(6,6);
A_des(1,1) = 1/(tau1_p*tau2_p*tau_des_p*tau3_p)*(-(tau3_p*tau_des_p*(tau1_p+tau2_p)+tau1_p*tau2_p*(tau_des_p+tau3_p)));
A_des(1,2) = 1/(tau1_p*tau2_p*tau_des_p*tau3_p)*(-(tau_des_p*tau3_p+tau1_p*tau2_p+tau_des_p*tau1_p+tau_des_p*tau2_p+tau3_p*tau1_p+tau3_p*tau2_p));
A_des(1,3) = 1/(tau1_p*tau2_p*tau_des_p*tau3_p)*(-(tau_des_p+tau1_p+tau2_p+tau3_p));
A_des(1,4) = -1/(tau1_p*tau2_p*tau_des_p*tau3_p);
A_des(2,1) = 1;
A_des(3,2) = 1;
A_des(4,3) = 1;
A_des(5,5) = -(tau3_q+tau_des_q)/(tau3_q*tau_des_q);
A_des(5,6) = -1/(tau3_q*tau_des_q);
A_des(6,5) = 1;  

Bh_des=zeros(6,2);
Bh_des(1,1) = 1/(tau1_p*tau2_p*tau_des_p*tau3_p);
Bh_des(5,2) = 1/(tau3_q*tau_des_q);

C_des = zeros(2,6);
C_des(1,1) = scaling3*(Mp_pu*theta1_p*tau3_p*tau2_p+Mp_pu*theta2_p*tau3_p*tau1_p-Mp_pu*tau1_p*tau2_p);
C_des(1,2) =scaling3*(Mp_pu*theta1_p*(tau3_p+tau2_p)+Mp_pu*theta2_p*(tau1_p+tau3_p)-Mp_pu*(tau1_p+tau2_p)+Dp_pu*theta1_p*tau3_p*tau2_p+Dp_pu*theta2_p*tau1_p*tau3_p-Dp_pu*tau1_p*tau2_p);
C_des(1,3) = scaling3*(Mp_pu*theta1_p+Mp_pu*theta2_p-Mp_pu+Dp_pu*theta1_p*(tau3_p+tau2_p)+Dp_pu*theta2_p*(tau1_p+tau3_p)-Dp_pu*(tau1_p+tau2_p));
C_des(1,4) = scaling3*(Dp_pu*theta1_p+Dp_pu*theta2_p-Dp_pu);
C_des(2,6) = scaling3*(-Dq1_pu*theta3_q);

Dh_des = zeros(2,2);

== matlab function CaseStudyII_9_Bus/STATCOM with Battery/Power Controllers1/DVPP State Feedback Controller/LPV Controller/MATLAB Function ==
  data: theta1_p input; theta2_p input; theta3_q input; theta1_p_1 input; theta1_p_2 input; lambda1 output; lambda2 output; theta2_p_1 input; theta2_p_2 input; lambda3 output; lambda4 output; theta3_q_1 input; theta3_q_2 input; lambda5 output; lambda6 output; lambda7 output; lambda8 output
function [lambda1,lambda2,lambda3,lambda4,lambda5,lambda6,lambda7,lambda8] = fcn(theta1_p,theta2_p,theta3_q,theta1_p_1,theta1_p_2,theta2_p_1,theta2_p_2,theta3_q_1,theta3_q_2)

lambda1 = ((theta1_p_2-theta1_p)*(theta2_p_2-theta2_p)*(theta3_q_2-theta3_q))/((theta1_p_2-theta1_p_1)*(theta2_p_2-theta2_p_1)*(theta3_q_2-theta3_q_1));
lambda2 = ((theta1_p_2-theta1_p)*(theta2_p-theta2_p_1)*(theta3_q_2-theta3_q))/((theta1_p_2-theta1_p_1)*(theta2_p_2-theta2_p_1)*(theta3_q_2-theta3_q_1));
lambda3 = ((theta1_p_2-theta1_p)*(theta2_p-theta2_p_1)*(theta3_q-theta3_q_1))/((theta1_p_2-theta1_p_1)*(theta2_p_2-theta2_p_1)*(theta3_q_2-theta3_q_1));
lambda4 = ((theta1_p_2-theta1_p)*(theta2_p_2-theta2_p)*(theta3_q-theta3_q_1))/((theta1_p_2-theta1_p_1)*(theta2_p_2-theta2_p_1)*(theta3_q_2-theta3_q_1));
lambda5 = ((theta1_p-theta1_p_1)*(theta2_p_2-theta2_p)*(theta3_q_2-theta3_q))/((theta1_p_2-theta1_p_1)*(theta2_p_2-theta2_p_1)*(theta3_q_2-theta3_q_1));
lambda6 = ((theta1_p-theta1_p_1)*(theta2_p-theta2_p_1)*(theta3_q_2-theta3_q))/((theta1_p_2-theta1_p_1)*(theta2_p_2-theta2_p_1)*(theta3_q_2-theta3_q_1));
lambda7 = ((theta1_p-theta1_p_1)*(theta2_p-theta2_p_1)*(theta3_q-theta3_q_1))/((theta1_p_2-theta1_p_1)*(theta2_p_2-theta2_p_1)*(theta3_q_2-theta3_q_1));
lambda8 = ((theta1_p-theta1_p_1)*(theta2_p_2-theta2_p)*(theta3_q-theta3_q_1))/((theta1_p_2-theta1_p_1)*(theta2_p_2-theta2_p_1)*(theta3_q_2-theta3_q_1));

== matlab function CaseStudyII_9_Bus/Wind /Power Controllers1/DVPP State Feedback Controller/MATLAB Function ==
  data: tau1_p input; tau1_q input; tau_des_p input; tau_des_q input; A_des output; scaling1 input; Bh_des output; C_des output; Dh_des output; theta1_p input; theta1_q input; Mp_pu input; Dp_pu input; Dq1_pu input
function [A_des, Bh_des, C_des, Dh_des] = fcn(tau1_p,tau1_q,tau_des_p,tau_des_q, scaling1, theta1_p, theta1_q, Mp_pu, Dp_pu, Dq1_pu)

%reference model at real-time measurement
A_des = zeros(4,4);
A_des(1,1)= -(tau1_p+tau_des_p)/(tau1_p*tau_des_p);
A_des(1,2)= -1/(tau1_p*tau_des_p);
A_des(2,1) = 1;
A_des(3,3)= -(tau1_q+tau_des_q)/(tau1_q*tau_des_q);
A_des(3,4)= -1/(tau1_q*tau_des_q);
A_des(4,3)=1;

Bh_des=zeros(4,2);
Bh_des(1,1) = 1/(tau1_p*tau_des_p);
Bh_des(3,2) = 1/(tau1_q*tau_des_q);

C_des = zeros(2,4);
C_des(1,1) = scaling1*(-theta1_p*Mp_pu);
C_des(1,2) =scaling1*(-theta1_p*Dp_pu);
C_des(2,4) = scaling1*(-theta1_q*Dq1_pu);

Dh_des = zeros(2,2);

== matlab function CaseStudyII_9_Bus/DVPP Operator /MATLAB Function ==
  data: S1 input; theta1_q output; S2 input; S3 input; P1 input; P2 input; P3 input; theta2_q output; theta3_q output
function [theta1_q,theta2_q,theta3_q] = fcn(S1,S2,S3,P1,P2,P3)

sum_sqrt = sqrt(S1^2-P1^2)+sqrt(S2^2-P2^2)+sqrt(S3^2-P3^2);
theta1_q = sqrt(S1^2-P1^2)/sum_sqrt;
theta2_q = sqrt(S2^2-P2^2)/sum_sqrt;
theta3_q = sqrt(S3^2-P3^2)/sum_sqrt;

== matlab function CaseStudyII_9_Bus/Wind /Power Controllers1/DVPP State Feedback Controller/LPV Controller/MATLAB Function ==
  data: theta1_p input; lambda1 output; theta1_q input; lambda2 output; theta1_p_1 input; theta1_p_2 input; theta1_q_1 input; theta1_q_2 input; lambda3 output; lambda4 output
function [lambda1,lambda2,lambda3,lambda4] = fcn(theta1_p,theta1_q,theta1_p_1, theta1_p_2, theta1_q_1, theta1_q_2)

%extreme points of the parameter polytope
a1_1 = [theta1_p_1; theta1_q_1];
a1_2 = [theta1_p_2; theta1_q_1];
a1_3 = [theta1_p_2; theta1_q_2];
a1_4 = [theta1_p_1; theta1_q_2];

lambda1 = ((theta1_p_2-theta1_p)*(theta1_q_2-theta1_q))/((theta1_p_2-theta1_p_1)*(theta1_q_2-theta1_q_1));
lambda2 = ((theta1_p-theta1_p_1)*(theta1_q_2-theta1_q))/((theta1_p_2-theta1_p_1)*(theta1_q_2-theta1_q_1));
lambda3 = ((theta1_p-theta1_p_1)*(theta1_q-theta1_q_1))/((theta1_p_2-theta1_p_1)*(theta1_q_2-theta1_q_1));
lambda4 = ((theta1_p_2-theta1_p)*(theta1_q-theta1_q_1))/((theta1_p_2-theta1_p_1)*(theta1_q_2-theta1_q_1));

== matlab function CaseStudyII_9_Bus/PV/Power Controllers/DVPP State Feedback Controller/MATLAB Function ==
  data: tau2_p input; tau2_q input; tau_des_p input; tau_des_q input; A_des output; scaling2 input; Bh_des output; C_des output; Dh_des output; theta2_p input; theta2_q input; Mp_pu input; Dp_pu input; Dq1_pu input
function [A_des, Bh_des, C_des, Dh_des] = fcn(tau2_p,tau2_q,tau_des_p,tau_des_q, scaling2, theta2_p, theta2_q, Mp_pu, Dp_pu, Dq1_pu)

%reference model at real-time measurement
A_des = zeros(4,4);
A_des(1,1)= -(tau2_p+tau_des_p)/(tau2_p*tau_des_p);
A_des(1,2)= -1/(tau2_p*tau_des_p);
A_des(2,1) = 1;
A_des(3,3)= -(tau2_q+tau_des_q)/(tau2_q*tau_des_q);
A_des(3,4)= -1/(tau2_q*tau_des_q);
A_des(4,3)=1;

Bh_des=zeros(4,2);
Bh_des(1,1) = 1/(tau2_p*tau_des_p);
Bh_des(3,2) = 1/(tau2_q*tau_des_q);

C_des = zeros(2,4);
C_des(1,1) = scaling2*(-theta2_p*Mp_pu);
C_des(1,2) =scaling2*(-theta2_p*Dp_pu);
C_des(2,4) = scaling2*(-theta2_q*Dq1_pu);

Dh_des = zeros(2,2);

== matlab function CaseStudyII_9_Bus/PV/Power Controllers/DVPP State Feedback Controller/LPV Controller/MATLAB Function ==
  data: theta2_p input; lambda1 output; theta2_q input; lambda2 output; theta2_p_1 input; theta2_p_2 input; theta2_q_1 input; theta2_q_2 input; lambda3 output; lambda4 output
function [lambda1,lambda2,lambda3,lambda4] = fcn(theta2_p,theta2_q,theta2_p_1, theta2_p_2, theta2_q_1, theta2_q_2)

lambda1 = ((theta2_p_2-theta2_p)*(theta2_q_2-theta2_q))/((theta2_p_2-theta2_p_1)*(theta2_q_2-theta2_q_1));
lambda2 = ((theta2_p-theta2_p_1)*(theta2_q_2-theta2_q))/((theta2_p_2-theta2_p_1)*(theta2_q_2-theta2_q_1));
lambda3 = ((theta2_p-theta2_p_1)*(theta2_q-theta2_q_1))/((theta2_p_2-theta2_p_1)*(theta2_q_2-theta2_q_1));
lambda4 = ((theta2_p_2-theta2_p)*(theta2_q-theta2_q_1))/((theta2_p_2-theta2_p_1)*(theta2_q_2-theta2_q_1));
